simulink model "model_controller"  (R2024a)
settings: Solver=FixedStepAuto  StartTime=0.0  StopTime=10.0  RelTol=1e-3
undefined symbols (not defined in the file or in its folder): A, ampl, B, Bw, C, Cz, Dw, Dz, K, phi, w
settings Model: Creator=anton  LastModifiedBy=anton

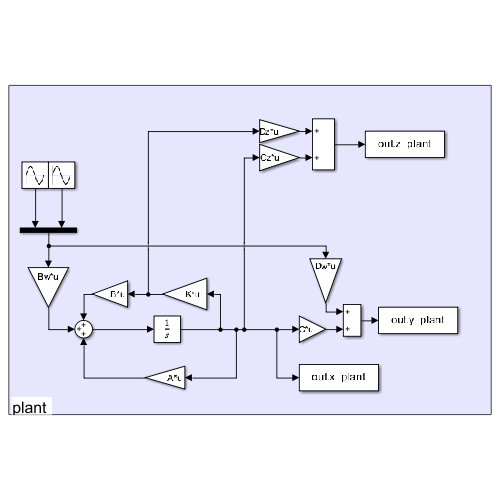
[thumbnail: Simulink's stored preview of the top-level diagram]
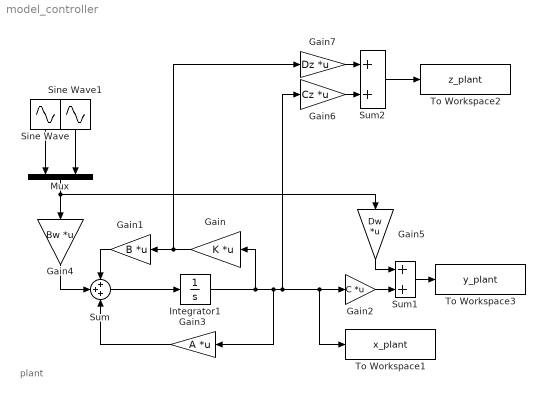
== system model_controller ==
  note: plant
  Gain : Gain  Gain=K  Multiplication=Matrix(K*u)
  Gain1 : Gain  Gain=B  Multiplication=Matrix(K*u)
  Gain2 : Gain  Gain=C  Multiplication=Matrix(K*u)
  Gain3 : Gain  Gain=A  Multiplication=Matrix(K*u)
  Gain4 : Gain  Gain=Bw  Multiplication=Matrix(K*u)
  Gain5 : Gain  Gain=Dw  Multiplication=Matrix(K*u)
  Gain6 : Gain  Gain=Cz  Multiplication=Matrix(K*u)
  Gain7 : Gain  Gain=Dz  Multiplication=Matrix(K*u)
  Integrator1 : Integrator
  Mux : Mux  Inputs=2
  Sine Wave : Sin  Amplitude=ampl  Frequency=w  Phase=phi  SampleTime=0
  Sine Wave1 : Sin  Amplitude=ampl  Frequency=w  Phase=phi  SampleTime=0
  Sum : Sum  Inputs=+++
  Sum1 : Sum
  Sum2 : Sum
  To Workspace1 : ToWorkspace  VariableName=x_plant  SaveFormat=Timeseries  SampleTime=-1
  To Workspace2 : ToWorkspace  VariableName=z_plant  SaveFormat=Timeseries  SampleTime=-1
  To Workspace3 : ToWorkspace  VariableName=y_plant  SaveFormat=Timeseries  SampleTime=-1
  wires:
  Integrator1/1 -> Gain/1, To Workspace1/1, Gain2/1, Gain6/1, Gain3/1
  Sum/1 -> Integrator1/1
  Gain/1 -> Gain7/1, Gain1/1
  Gain1/1 -> Sum/1
  Gain3/1 -> Sum/3
  Gain4/1 -> Sum/2
  Gain2/1 -> Sum1/2
  Sum1/1 -> To Workspace3/1
  Gain5/1 -> Sum1/1
  Sum2/1 -> To Workspace2/1
  Gain6/1 -> Sum2/2
  Gain7/1 -> Sum2/1
  Sine Wave/1 -> Mux/1
  Sine Wave1/1 -> Mux/2
  Mux/1 -> Gain5/1, Gain4/1
